simulink model "PlantaOficial"  (R2024b)
settings: Solver=ode23tb  StartTime=0.0  StopTime=39  RelTol=1e-3
values from neighbouring files (symbols this model uses):
  C1 = 1.2801    [CodigoSavePoint.m]    (also in CodigoVT.m)
  C2 = 23.99    [CodigoSavePoint.m]    (also in CodigoVT.m)
  C3 = 0.52    [CodigoSavePoint.m]    (also in CodigoVT.m)
  VelRef = 17    [CodigoSavePoint.m]    (also in CodigoVT.m = 30)
undefined symbols (not defined in the file or in its folder): EV, fractalcoef, MTR
libraries: autolibmappedmotor x2, vrlib x1, slpidlib x1, mspsensorlib x1, vehdynlibviscommon x1, vehdynlibtire x1, vehdynlibscenariocommon x1, vehdynlibsteering x1, vehdynlibdriver x1, autolibshared x1
(part 1 of 2)
settings Model: Creator=João Gabriel  LastModifiedBy=João Gabriel

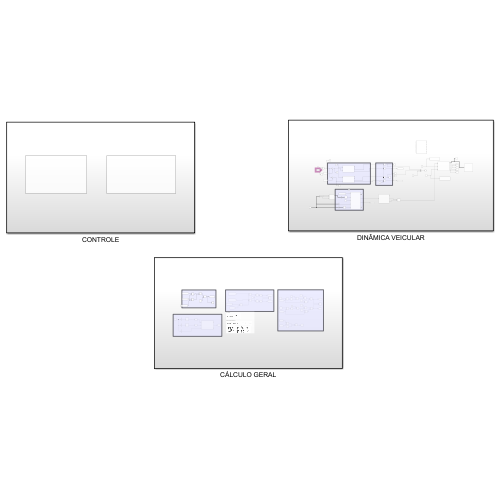
[thumbnail: Simulink's stored preview of the top-level diagram]
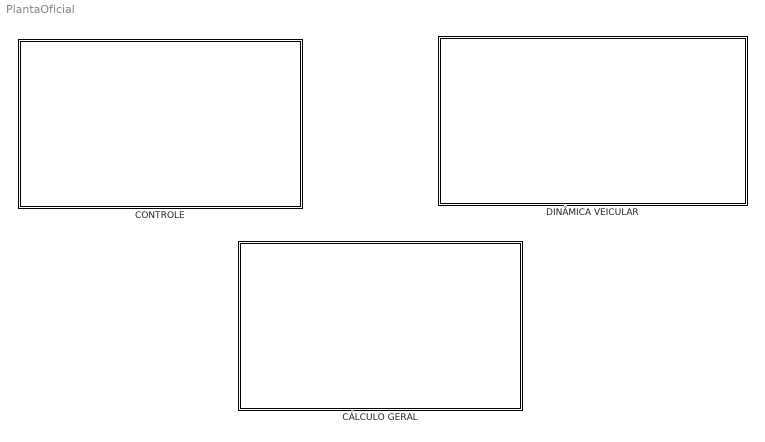
== system PlantaOficial ==
  CONTROLE : Subsystem
  CÁLCULO GERAL : Subsystem
  DINÂMICA VEICULAR : Subsystem

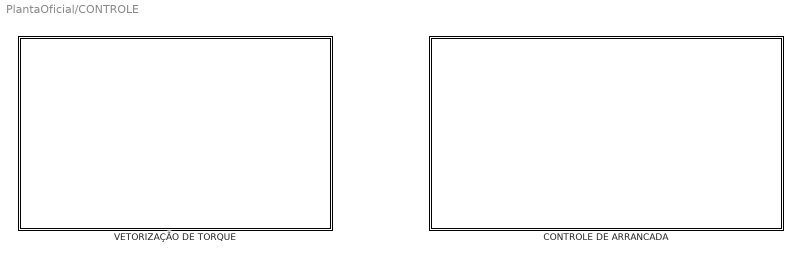
== system PlantaOficial/CONTROLE ==
  "CONTROLE DE ARRANCADA " : Subsystem
  "VETORIZAÇÃO DE TORQUE " : Subsystem

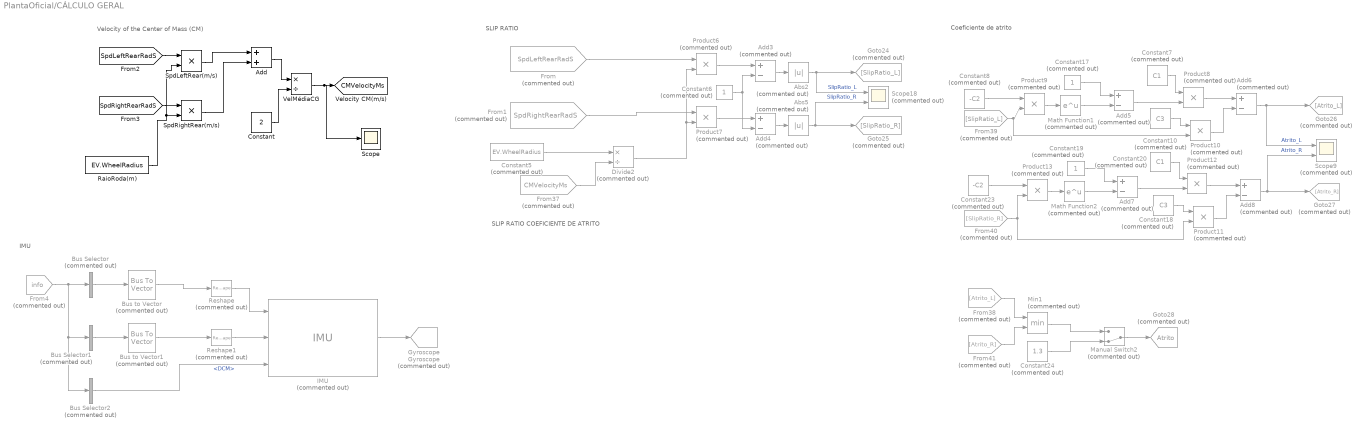
== system PlantaOficial/CÁLCULO GERAL ==
  note: IMU
  note: Velocity of the Center of Mass (CM)
  note: SLIP RATIO
  note: Coeficiente de atrito
  note: SLIP RATIO
      |
      | COEFICIENTE DE ATRITO
  Abs2 : Abs  Commented=on  SaturateOnIntegerOverflow=off
  Abs5 : Abs  Commented=on  SaturateOnIntegerOverflow=off
  Add : Sum
  Add{3..8} (6 alike) : Sum  Commented=on  Inputs=+-
  Bus Selector : BusSelector  Commented=on  OutputSignals=BdyFrm.Cg.Acc.zddot,BdyFrm.Cg.Acc.yddot,BdyFrm.Cg.Acc.xddot  OutputAsBus=on
  Bus Selector1 : BusSelector  Commented=on  OutputSignals=BdyFrm.Cg.AngVel.p,BdyFrm.Cg.AngVel.q,BdyFrm.Cg.AngVel.r  OutputAsBus=on
  Bus Selector2 : BusSelector  Commented=on  OutputSignals=BdyFrm.Cg.DCM
  Bus to Vector : BusToVector  Commented=on
  Bus to Vector1 : BusToVector  Commented=on
  Constant : Constant  Value=2
  Constant10 : Constant  Commented=on  Value=C3
  Constant17 : Constant  Commented=on
  Constant18 : Constant  Commented=on  Value=C3
  Constant19 : Constant  Commented=on
  Constant20 : Constant  Commented=on  Value=C1
  Constant23 : Constant  Commented=on  Value=-C2
  Constant24 : Constant  Commented=on  Value=1.3  VectorParams1D=off
  Constant5 : Constant  Commented=on  Value=EV.WheelRadius  VectorParams1D=off
  Constant6 : Constant  Commented=on
  Constant7 : Constant  Commented=on  Value=C1
  Constant8 : Constant  Commented=on  Value=-C2
  Divide2 : Product  Commented=on  Inputs=*/
  From : From  Commented=on  GotoTag=SpdLeftRearRadS  TagVisibility=global
  From1 : From  Commented=on  GotoTag=SpdRightRearRadS  TagVisibility=global
  From37 : From  Commented=on  GotoTag=CMVelocityMs  TagVisibility=global
  From38 : From  Commented=on  GotoTag=Atrito_L
  From39 : From  Commented=on  GotoTag=SlipRatio_L
  From4 : From  Commented=on  GotoTag=info  TagVisibility=global
  From40 : From  Commented=on  GotoTag=SlipRatio_R
  From41 : From  Commented=on  GotoTag=Atrito_R
  Goto24 : Goto  Commented=on  GotoTag=SlipRatio_L
  Goto25 : Goto  Commented=on  GotoTag=SlipRatio_R
  Goto26 : Goto  Commented=on  GotoTag=Atrito_L
  Goto27 : Goto  Commented=on  GotoTag=Atrito_R
  Goto28 : Goto  Commented=on  GotoTag=Atrito  TagVisibility=global
  "Gyroscope " : Goto  Commented=on  GotoTag=Gyroscope  TagVisibility=global
  IMU : mspsensorlib/IMU  Commented=on  DispRefFrame=NED  TemperaturePort=off  Temperature=25  MagneticFieldPort=off  MagneticFieldNED=[ 27.5550, -2.4169, -16.0849 ]  MagneticFieldENU=[ -2.4169, 27.5550, 16.0849 ]  SeedDouble=67  SimulateUsing=Interpreted execution  AccelParamsMeasurementRange=Inf  AccelParamsResolution=0  AccelParamsConstantBias=[ 0, 0, 0 ]  AccelParamsAxesMisalignment=[ 100, 0, 0; 0, 100, 0; 0, 0, 100 ]  AccelParamsNoiseDensity=[ 0, 0, 0 ]  AccelParamsBiasInstability=[ 0, 0, 0 ]  AccelParamsBiasInstabilityNumerator=fractalcoef().Numerator  AccelParamsBiasInstabilityDenominator=fractalcoef().Denominator  AccelParamsRandomWalk=[ 0, 0, 0 ]  AccelParamsNoiseType=double-sided  AccelParamsTemperatureBias=[ 0, 0, 0 ]  AccelParamsTemperatureScaleFactor=[ 0, 0, 0 ]  GyroParamsMeasurementRange=Inf  GyroParamsResolution=0  GyroParamsConstantBias=[ 0, 0, 0 ]  GyroParamsAxesMisalignment=[ 100, 0, 0; 0, 100, 0; 0, 0, 100 ]  GyroParamsAccelerationBias=[ 0, 0, 0 ]  GyroParamsNoiseDensity=[ 0, 0, 0 ]  GyroParamsBiasInstability=[ 0, 0, 0 ]  GyroParamsBiasInstabilityNumerator=fractalcoef().Numerator  GyroParamsBiasInstabilityDenominator=fractalcoef().Denominator  GyroParamsRandomWalk=[ 0, 0, 0 ]  GyroParamsNoiseType=double-sided  GyroParamsTemperatureBias=[ 0, 0, 0 ]  GyroParamsTemperatureScaleFactor=[ 0, 0, 0 ]  MagParamsMeasurementRange=Inf  MagParamsResolution=0  MagParamsConstantBias=[ 0, 0, 0 ]  MagParamsAxesMisalignment=[ 100, 0, 0; 0, 100, 0; 0, 0, 100 ]  MagParamsNoiseDensity=[ 0, 0, 0 ]  MagParamsBiasInstability=[ 0, 0, 0 ]  MagParamsBiasInstabilityNumerator=fractalcoef().Numerator  MagParamsBiasInstabilityDenominator=fractalcoef().Denominator  MagParamsRandomWalk=[ 0, 0, 0 ]  MagParamsNoiseType=double-sided  MagParamsTemperatureBias=[ 0, 0, 0 ]  MagParamsTemperatureScaleFactor=[ 0, 0, 0 ]
  Manual Switch2 : ManualSwitch  Commented=on  CurrentSetting=0
  Math Function1 : Math  Commented=on
  Math Function2 : Math  Commented=on
  Min1 : MinMax  Commented=on  Inputs=2
  Product{6..13} (8 alike) : Product  Commented=on
  RaioRoda(m) : Constant  Value=EV.WheelRadius  VectorParams1D=off
  Reshape : Reshape  Commented=on  OutputDimensionality=Customize  OutputDimensions=[1,3]
  Reshape1 : Reshape  Commented=on  OutputDimensionality=Customize  OutputDimensions=[1,3]
  Scope : Scope
  Scope18 : Scope  Commented=on  NumInputPorts=2
  Scope9 : Scope  Commented=on  NumInputPorts=2
  SpdLeftRear(m/s) : Product
  SpdRightRear(m/s) : Product
  VelMédiaCG : Product  Inputs=*/
  tag scope: CMVelocityMs=global
  wires:
  Constant6/1 -> Add3/2, Add4/2
  Add6/1 -> Scope9/1, Goto26/1  "Atrito_L"
  Abs2/1 -> Scope18/1, Goto24/1  "SlipRatio_L"
  Constant7/1 -> Product8/1
  Constant19/1 -> Add7/1
  Constant24/1 -> Manual Switch2/2
  Constant23/1 -> Product13/1
  Add4/1 -> Abs5/1
  Add3/1 -> Abs2/1
  Product11/1 -> Add8/2
  Abs5/1 -> Scope18/2, Goto25/1  "SlipRatio_R"
  Product12/1 -> Add8/1
  Product10/1 -> Add6/2
  Product8/1 -> Add6/1
  Math Function2/1 -> Add7/2
  Add7/1 -> Product12/2
  From38/1 -> Min1/1
  Constant10/1 -> Product10/1
  Math Function1/1 -> Add5/2
  Constant18/1 -> Product11/1
  From39/1 -> Product10/2, Product9/2
  Add8/1 -> Scope9/2, Goto27/1  "Atrito_R"
  Product9/1 -> Math Function1/1
  From37/1 -> Divide2/2
  Min1/1 -> Manual Switch2/1
  Constant8/1 -> Product9/1
  Constant17/1 -> Add5/1
  From41/1 -> Min1/2
  Constant5/1 -> Divide2/1
  Divide2/1 -> Product6/2, Product7/2
  Product13/1 -> Math Function2/1
  Constant20/1 -> Product12/1
  Product7/1 -> Add4/1
  Add5/1 -> Product8/2
  From40/1 -> Product13/2, Product11/2
  Product6/1 -> Add3/1
  Manual Switch2/1 -> Goto28/1
  From1/1 -> Product7/1
  From/1 -> Product6/1
  Add/1 -> VelMédiaCG/1
  RaioRoda(m)/1 -> SpdLeftRear(m/s)/2, SpdRightRear(m/s)/2
  Constant/1 -> VelMédiaCG/2
  SpdLeftRear(m/s)/1 -> Add/1
  SpdRightRear(m/s)/1 -> Add/2
  [SpdLeftRearRadS] -> SpdLeftRear(m/s)/1
  [SpdRightRearRadS] -> SpdRightRear(m/s)/1
  VelMédiaCG/1 -> Scope/1, [CMVelocityMs]
  From4/1 -> Bus Selector2/1, Bus Selector1/1, Bus Selector/1
  Bus Selector2/1 -> IMU/3  "<DCM>"
  IMU/2 -> "Gyroscope "/1
  Bus Selector/1 -> Bus to Vector/1
  Bus to Vector/1 -> Reshape/1
  Reshape/1 -> IMU/1
  Bus Selector1/1 -> Bus to Vector1/1
  Bus to Vector1/1 -> Reshape1/1
  Reshape1/1 -> IMU/2

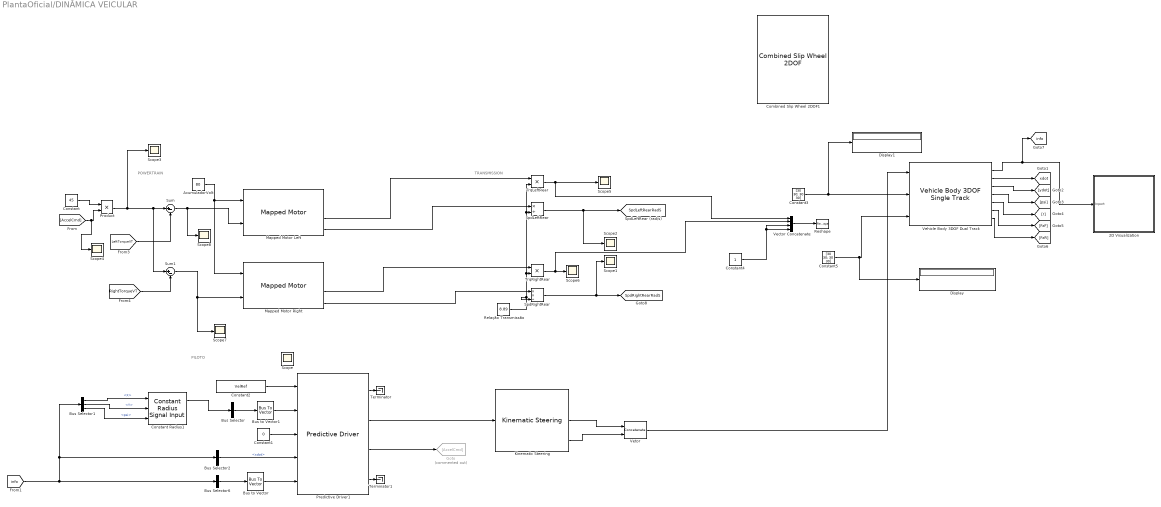
== system PlantaOficial/DINÂMICA VEICULAR ==
  note: TRANSMISSION
  note: POWERTRAIN
  note: PILOTO
  2D Visualization : Subsystem
      mask Display: image("visualization.JPG");
  AcumuladorVolt : Constant  Value=80
  Bus Selector : BusSelector  OutputSignals=XRef,YRef,PhiRef  OutputAsBus=on
  Bus Selector1 : BusSelector  OutputSignals=InertFrm.Cg.Disp.X,InertFrm.Cg.Disp.Y,InertFrm.Cg.Ang.psi
  Bus Selector2 : BusSelector  OutputSignals=BdyFrm.Cg.Vel.xdot
  Bus Selector6 : BusSelector  OutputSignals=InertFrm.Cg.Disp.X,InertFrm.Cg.Disp.Y,InertFrm.Cg.Disp.Z  OutputAsBus=on
  Bus to Vector : BusToVector
  Bus to Vector1 : BusToVector
  Combined Slip Wheel 2DOF1 : vehdynlibtire/Combined Slip Wheel 2DOF  tireType=Mid-size passenger car 235/45R18  tireParamSet=vdynPassCar.mat  vertType=Magic Formula  plySteer=on  turnslip=off  BrakeType=Disc  mu_static=.3  mu_kinetic=.2  drum_abore=0.0508  drum_a=0.123  drum_c=0.212  drum_r=0.15  drum_theta1=0  drum_theta2=126  disk_abore=.05  Rm=.177  num_pads=2  brake_p_bpt=[1 11.4736842105263 21.9473684210526 32.4210526315789 42.8947368421053 53.3684210526316 63.8421052631579 74.3157894736842 84.7894736842105 95.2631578947368 105.736842105263 116.210526315789 126.684210526316 137.157894736842 147.631578947368 158.105263157895 168.578947368421 179.052631578947 189.526315789474 200]  brake_n_bpt=[0 52.6315789473684 105.263157894737 157.894736842105 210.526315789474 263.157894736842 315.789473684211 368.421052631579 421.052631578947 473.684210526316 526.315789473684 578.947368421053 631.578947368421 684.210526315789 736.842105263158 789.473684210526 842.105263157895 894.736842105263 947.368421052632 1000]  f_brake_t=[43.4900602404453 42.5056030554862 41.5350898940194 40.5780454442085 39.6340111501808 38.7025443887544 37.7832176914519 36.8756180088306 35.9793460143796 35.0940154454303 34.2192524787115 33.3546951383474 32.4999927342521 31.6548053290159 30.8188032315107 29.991666515561 29.1730845621415 28.362755623661 27.5603864089927 26.765691687993;498.991217495636 487.695866636631 476.560505099801 465.579679307235 454.748127933653 444.060772460445 433.51270824929 423.099196101319 412.81565427025 402.657650900201 392.620896861006 382.701238955775 372.894653477208 363.197240090814 353.605216024701 344.114910546964 334.722759712992 325.425301366216 316.219170376863 307.10109410434;954.492374750826 932.886130217776 911.585920305583 890.581313170261 869.862244717126 849.419000532136 829.242198807128 809.322774193808 789.651962526121 770.221286354971 751.0225412433 732.047782773203 713.289314220164 694.739674852612 676.391628817892 658.238154578366 640.272434863842 622.48784710877 604.877954344734 587.436496520688;1409.99353200602 1378.07639379892 1346.61133551136 1315.58294703329 1284.9763615006 1254.77722860383 1224.97168936497 1195.5463522863 1166.48827078199 1137.78492180974 1109.42418562559 1081.39432659063 1053.68397496312 1026.28210961441 999.178041611083 972.361398609768 945.822110014692 919.550392851325 893.536738312604 867.771898937035;1865.49468926121 1823.26665738007 1781.63675071715 1740.58458089631 1700.09047828407 1660.13545667552 1620.7011799228 1581.76993037878 1543.32457903786 1505.34855726451 1467.82583000789 1430.74087040806 1394.07863570608 1357.82454437621 1321.96445440427 1286.48464264117 1251.37178516554 1216.61293859388 1182.19552228048 1148.10730135338;2320.9958465164 2268.45692096121 2216.66216592293 2165.58621475934 2115.20459506754 2065.49368474721 2016.43067048064 1967.99350847127 1920.16088729373 1872.91219271928 1826.22747439018 1780.08741422549 1734.47329644903 1689.36697913801 1644.75086719747 1600.60788667257 1556.92146031639 1513.67548433643 1470.85430624835 1428.44270376973;2776.49700377159 2713.64718454235 2651.68758112871 2590.58784862237 2530.31871185102 2470.8519128189 2412.16016103848 2354.21708656376 2296.9971955496 2240.47582817405 2184.62911877248 2129.43395804292 2074.86795719199 2020.9094138998 1967.53727999066 1914.73113070398 1862.47113546724 1810.73803007899 1759.51309021622 1708.77810618608;3231.99816102678 3158.8374481235 3086.71299633449 3015.58948248539 2945.43282863449 2876.21014089059 2807.88965159632 2740.44066465625 2673.83350380547 2608.03946362882 2543.03076315477 2478.78050186034 2415.26261793494 2352.4518486616 2290.32369278385 2228.85437473538 2168.02081061809 2107.80057582154 2048.17187418409 1989.11350860242;3687.49931828197 3604.02771170464 3521.73841154027 3440.59111634842 3360.54694541796 3281.56836896228 3203.61914215416 3126.66424274874 3050.66981206134 2975.60309908359 2901.43240753707 2828.12704567777 2755.6572786779 2683.9942834234 2613.11010557704 2542.97761876678 2473.57048576894 2404.8631215641 2336.83065815196 2269.44891101877;4143.00047553716 4049.21797528579 3956.76382674606 3865.59275021144 3775.66106220143 3686.92659703397 3599.34863271199 3512.88782084123 3427.50612031721 3343.16673453836 3259.83405191936 3177.4735894952 3096.05193942085 3015.5367181852 2935.89651837023 2857.10086279818 2779.12016091979 2701.92566730665 2625.48944211983 2549.78431343512;4598.50163279235 4494.40823886693 4391.78924195184 4290.59438407447 4190.77517898491 4092.28482510566 3995.07812326983 3899.11139893372 3804.34242857308 3710.73036999313 3618.23569630166 3526.82013331263 3436.44660016381 3347.079152947 3258.68293116342 3171.22410682959 3084.66983607064 2998.98821304921 2914.1482260877 2830.11971585147;5054.00279004754 4939.59850244808 4826.81465715762 4715.59601793749 4605.88929576838 4497.64305317735 4390.80761382767 4285.3349770262 4181.17873682896 4078.2940054479 3976.63734068395 3876.16667713006 3776.84126090677 3678.62158770879 3581.46934395661 3485.34735086099 ...(+2764 chars)]  NOMPRES=262000  PRESMAX=1000000  PRESMIN=10000  FNOMIN=4300  FZMAX=8600  FZMIN=100  VXLOW=1  KPUMAX=1.5  KPUMIN=-1.5  ALPMAX=1.5  ALPMIN=-1.5  CAMMAX=0.17453  CAMMIN=-0.17453  LONGVL=16.7  FxRelFreqLwrLim=200*pi  FyRelFreqLwrLim=200*pi  MyRelFreqLwrLim=100*pi  omegao=0  UNLOADED_RADIUS=0.33454  WIDTH=0.235  RIM_RADIUS=0.2286  ASPECT_RATIO=0.45  MASS=11.2  IYY=1.084  br=1e-3  GRAVITY=-9.81  zo=0  zdoto=0  BREFF=8.25094594147963  DREFF=0.260468730454265  FREFF=0.0735298544471851  Q_RE0=1.00866439868088  Q_V1=0.000760413786224011  Q_V2=0.0463384792019201  Q_FZ1=0  Q_FZ2=15.6870832810226  Q_FZ3=0  Q_FCX=0.138643970247602  Q_FCY=0.10843499565426  Q_FCY2=-0.465763352339538  PFZ1=0.69958166705601  VERTICAL_STIFFNESS=207885.061134007  VERTICAL_DAMPING=500  BOTTOM_OFFST=0.00990653336182505  BOTTOM_STIFF=1999075.87051971  Q_CAM1=86.7791723017291  Q_CAM2=259.705254231766  Q_CAM3=0.510281667378416  Q_FYS1=-20769.4728880343  Q_FYS2=-59060.183485617  Q_FYS3=89271.8260126986  LONGITUDINAL_STIFFNESS=388714.175879854  LATERAL_STIFFNESS=157087.404633332  PCFX1=0.18539229191199  PCFX2=0  PCFX3=0  PCFY1=0.163183345037677  PCFY2=0  PCFY3=0.249094918231954  Q_RA1=0.675942571700787  Q_RA2=0.73800463546164  Q_RB1=1.04487486456705  Q_RB2=-1.191763806629  PCX1=1.58523057950359  PDX1=1.0239116238178  PDX2=-0.0842405110022724  PDX3=0  PEX1=0.110312777158455  PEX2=0.313468516038146  PEX3=0  PEX4=0.0016060905760045  PKX1=21.3872544684023  PKX2=14.0006541873175  PKX3=-0.405326109653452  PHX1=0.000212599305364818  PHX2=0.00115950515263055  PVX1=1.59236164471432e-05  PVX2=0.000104321112127671  PPX1=-0.349461321276586  PPX2=0.387840040616429  PPX3=-0.0969947336569324  PPX4=0.0632271859795801  RBX1=12.7633329850276  RBX2=9.5787123658471  RBX3=0  RCX1=1.02796280922059  REX1=-0.45202516851367  REX2=-0.47304886171176  RHX1=0.000233272373115809  QSX1=-0.00788307788961443  QSX2=0.954629515459396  QSX3=0.0155855777667025  QSX4=0.125904607142414  QSX5=1.01110069703963  QSX6=20.1938577118433  QSX7=0.310818120717083  QSX8=-0.0430823751139655  QSX9=0.636494404888216  QSX10=0.142438060591663  QSX11=0.346766530036373  QSX12=0  QSX13=0  QSX14=0  PPMX1=0  PCY1=1.34299950037631  PDY1=0.878267729082195  PDY2=-0.0644597923147385  PDY3=0  PEY1=-0.809776534470972  PEY2=-0.600180598867198  PEY3=0.0991732552633487  PEY4=-6.5577974035573  PEY5=0  PKY1=-15.5714726518315  PKY2=1.73126522291751  PKY3=0.365349873517229  PKY4=1.98176755955416  PKY5=0  PKY6=-0.884005199550313  PKY7=-0.237259727611847  PHY1=-0.00183370557235628  PHY2=0.00346401302716671  PVY1=-0.00675427560163264  PVY2=0.036379218103843  PVY3=-0.163543984089166  PVY4=-0.491003349625726  PPY1=-0.62059646553185  PPY2=-0.0647824842338686  PPY3=-0.164648843290686  PPY4=0.283193909060098  PPY5=0  RBY1=10.7588809173639  RBY2=7.70420065295029  RBY3=3.40283755070691e-06  RBY4=0  RCY1=1.06691874059059  REY1=0.308244924574305  REY2=7.48775032604508e-06  RHY1=0.0118479204960415  RHY2=7.63650177161071e-06  RVY1=0.0560024425050078  RVY2=7.48487127056197e-06  RVY3=0  RVY4=98.4047026517149  RVY5=2.02759273900054  RVY6=15.7623064923347  QSY1=0.00699077564863536  QSY2=0  QSY3=0.00153535478298811  QSY4=8.55710322455322e-05  QSY5=0  QSY6=0  QSY7=0.89443879773793  QSY8=-0.403227641260894  QBZ1=11.666656027484  QBZ2=-1.30355438574485  QBZ3=0  QBZ4=0.177918305399071  QBZ5=-0.162481135068033  QBZ6=0  QBZ9=30.1445534682089  QBZ10=0  QCZ1=1.29026978207574  QDZ1=0.0886972644991399  QDZ2=-0.0058634820161856  QDZ3=0.3805597481383  QDZ4=0  QDZ6=0.00160914918118959  QDZ7=-0.00211036330862154  QDZ8=-0.13921904912557  QDZ9=0.00816585550028243  QDZ10=0  QDZ11=0  QEZ1=-2.19802254534746  QEZ2=1.01850535789165  QEZ3=0  QEZ4=0.278379679112054  QEZ5=-0.548414722765386  QHZ1=0.00148361198869669  QHZ2=0.00202017567585904  QHZ3=0.240316641332066  QHZ4=-0.210114035738085  PPZ1=-0.443927982388615  PPZ2=0  SSZ1=0.00914999585397887  SSZ2=0.0389830656052735  SSZ3=0  SSZ4=0  PDXP1=0.396718274678791  PDXP2=0  PDXP3=0  PKYP1=1.00587060633573  PDYP1=0.40483048923438  PDYP2=0  PDYP3=0  PDYP4=0  PHYP1=0.992731942067188  PHYP2=0.150352945499914  PHYP3=0  PHYP4=-3.98988682633674  PECP1=0.502379254513503  PECP2=0  QDTP1=10.0178654287947  QCRP1=0.200627747200702  QCRP2=0.0995735881599772  QBRP1=0.0997107127960717  QDRP1=1.01432910167423  QDRP2=0  aMode=2
  Constant : Constant  Value=45  VectorParams1D=off
  Constant Radius1 : vehdynlibscenariocommon/Constant Radius Signal Input  VariantControl=4  tStart=0  velRef=VelRef  velRefUnit=m/s  R=50  X_o=0  Y_o=0  psi_o=0  radialConeDist=6  ayMax=0.5  steerDir=Right  ayStop=off  use3DCones=off  aMode=2
      settings: LibrarySourceBlock=vehdynlibscenario/Constant Radius
  Constant1 : Constant  Value=0
  Constant2 : Constant  Value=VelRef  VectorParams1D=off
  Constant3 : Constant  Value=[30 30; 30 30]
  Constant4 : Constant
  Constant5 : Constant  Value=[30 30; 30 30]
  Display : Display
  Display1 : Display
  Goto : Goto  Commented=on  GotoTag=AccelCmd
  Kinematic Steering : vehdynlibsteering/Kinematic Steering  StrgType=Rack and pinion  StrgRatioType=Constant  Loc=Front  NrmlFctr=0.01  TrckWdth=1  WhlBase=1.524  Db=0  StrgRng=1.25*pi  StrgAngBpts="[-6.2832   -5.0265   -3.7699   -2.5133   -1.2566         0    1.2566    2.5133    3.7699    5.0265    6.2832]"  StrgRatioTbl=|  StrgRatio=100  PctAckIn=off  PctAck=100  PctAckTbl=ones(1,11)*100  StrgArmLngth=0.1  RckCsLngth=0.5  TieRodLngth=0.248  D=0.2  PnnRadius=0.00085818  PnnRadiusTbl="[0.0055    0.0055    0.0056    0.0057    0.0058    0.0057    0.0057    0.0057    0.0056    0.0055    0.0055]"  RodLngth=0.1  ParaArmLngth=0.9  aMode=2
      | [13.5000   13.3750   13.2500   13.1250   13.0000   13.0000   13.0000   13.1250   13.2500   13.3750   13.5000
      | ]
  Mapped Motor Left : autolibmappedmotor/Mapped Motor  w_Tmax_bp_ext=w_Tmax_bp  Tmax_w_V_ext=Tmax_w_V  w_Tmin_bp_ext=w_Tmin_bp  Tmin_w_V_ext=Tmin_w_V  port_config=Torque  param_by=Tabulated torque-speed envelope  w_t=MTR.Speed  T_t=MTR.Torque*MTR.Overpower  torque_max=.1  power_max=30  SpreadsheetTqLimitsFileName=MotorCalibrationImportData.xlsx  Tmax_w_V=[0.09 0.09 0.09;0.08 0.08 0.08;0.07 0.07 0.07;0 0 0]  w_Tmax_bp=[ 0 375 750 800 ]  V_Tmax_bp=[500 750 900]  Tmin_w_V=[-0.09 -0.09 -0.09;-0.08 -0.08 -0.08;-0.07 -0.07 -0.07;0 0 0]  w_Tmin_bp=[ 0 375 750 800 ]  V_Tmin_bp=[500 750 900]  Tc=0.05  param_loss=Single efficiency measurement  SpreadsheetLossFileName=MotorCalibrationImportData.xlsx  SpreadsheetEffFileName=MotorCalibrationImportData.xlsx  eff=100  w_eff=375  T_eff=0.08  Piron=0  Pbase=0  w_eff_bp=[-8000 -4000 0 4000 8000]  T_eff_bp=[0 0.03 0.06 0.09]  Temp_eff_bp=[233.15 293.15 373.15]  V_eff_bp=[500 700 900]  losses_table=[1.49 1.67 2.21 3.10; 0.42 0.69 1.14 2.03; 0.06 0.24 0.78 1.68; 0.42 0.69 1.14 2.03; 1.49 1.67 2.21 3.10]  losses_table_3d=cat(3,1.05*[1.49 1.67 2.21 3.10; 0.42 0.69 1.14 2.03; 0.06 0.24 0.78 1.68; 0.42 0.69 1.14 2.03; 1.49 1.67 2.21 3.10],[1.49 1.67 2.21 3.10; 0.42 0.69 1.14 2.03; 0.06 0.24 0.78 1.68; 0.42 0.69 1.14 2.03; 1.49 1.67 2.21 3.10],1.03*[1.49 1.67 2.21 3.10; 0.42 0.69 1.14 2.03; 0.06 0.24 0.78 1.68; 0.42 0.69 1.14 2.03; 1.49 1.67 2.21 3.10])  losses_table_4d=cat(4,cat(3,[1.5645 0.441 0.063 0.441 1.5645;1.7535 0.7245 0.252 0.7245 1.7535;2.3205 1.197 0.819 1.197 2.3205;3.255 2.1315 1.764 2.1315 3.255],[1.5645 0.441 0.063 0.441 1.5645;1.7535 0.7245 0.252 0.7245 1.7535;2.3205 1.197 0.819 1.197 2.3205;3.255 2.1315 1.764 2.1315 3.255],[1.5645 0.441 0.063 0.441 1.5645;1.7535 0.7245 0.252 0.7245 1.7535;2.3205 1.197 0.819 1.197 2.3205;3.255 2.1315 1.764 2.1315 3.255]),cat(3,[1.49 0.42 0.06 0.42 1.49;1.67 0.69 0.24 0.69 1.67;2.21 1.14 0.78 1.14 2.21;3.1 2.03 1.68 2.03 3.1],[1.49 0.42 0.06 0.42 1.49;1.67 0.69 0.24 0.69 1.67;2.21 1.14 0.78 1.14 2.21;3.1 2.03 1.68 2.03 3.1],[1.49 0.42 0.06 0.42 1.49;1.67 0.69 0.24 0.69 1.67;2.21 1.14 0.78 1.14 2.21;3.1 2.03 1.68 2.03 3.1]),cat(3,[1.5347 0.4326 0.0618 0.4326 1.5347;1.7201 0.7107 0.2472 0.7107 1.7201;2.2763 1.1742 0.8034 1.1742 2.2763;3.193 2.0909 1.7304 2.0909 3.193],[1.5347 0.4326 0.0618 0.4326 1.5347;1.7201 0.7107 0.2472 0.7107 1.7201;2.2763 1.1742 0.8034 1.1742 2.2763;3.193 2.0909 1.7304 2.0909 3.193],[1.5347 0.4326 0.0618 0.4326 1.5347;1.7201 0.7107 0.2472 0.7107 1.7201;2.2763 1.1742 0.8034 1.1742 2.2763;3.193 2.0909 1.7304 2.0909 3.193]))  efficiency_table=[95 95 95 95; 95 95 95 95; 95 95 95 95; 95 95 95 95; 95 95 95 95]  efficiency_table_3d=cat(3,90*ones(5,4),95*ones(5,4),92*ones(5,4))  efficiency_table_4d=cat(4,cat(3,90*ones(5,4)',90*ones(5,4)',90*ones(5,4)'),cat(3,95*ones(5,4)',95*ones(5,4)',95*ones(5,4)'),cat(3,92*ones(5,4)',92*ones(5,4)',92*ones(5,4)'))  J=5e-6  b=1e-5  omega_o=0  T_t_extended=[0.35 22.4 23.8 26.95 31.5 37.1 45.85 45.85 45.85 37.1 31.5 26.95 23.8 22.4 0.35]  w_t_extended=[-943 -942 -880 -775 -670 -565 -461 0 461 565 670 775 880 942 943]  KLossIron=0  KLossCopper=0  x_w_eff_vec=[-8000 -4000 0 4000 8000]  x_T_eff_vec=[-0.09 -0.06 -0.03 0 0.03 0.06 0.09]  x_tmp_eff_vec=[233.15 293.15 373.15]  x_V_eff_vec=[500 700 900]  x_losses_mat=[3.1 2.21 1.67 1.49 1.67 2.21 3.1;2.03 1.14 0.69 0.42 0.69 1.14 2.03;1.68 0.78 0.24 0.06 0.24 0.78 1.68;2.03 1.14 0.69 0.42 0.69 1.14 2.03;3.1 2.21 1.67 1.49 1.67 2.21 3.1]  x_losses_mat_3d=cat(3,[3.255 2.3205 1.7535 1.5645 1.7535 2.3205 3.255;2.1315 1.197 0.7245 0.441 0.7245 1.197 2.1315;1.764 0.819 0.252 0.063 0.252 0.819 1.764;2.1315 1.197 0.7245 0.441 0.7245 1.197 2.1315;3.255 2.3205 1.7535 1.5645 1.7535 2.3205 3.255],[3.1 2.21 1.67 1.49 1.67 2.21 3.1;2.03 1.14 0.69 0.42 0.69 1.14 2.03;1.68 0.78 0.24 0.06 0.24 0.78 1.68;2.03 1.14 0.69 0.42 0.69 1.14 2.03;3.1 2.21 1.67 1.49 1.67 2.21 3.1],[3.193 2.2763 1.7201 1.5347 1.7201 2.2763 3.193;2.0909 1.1742 0.7107 0.4326 0.7107 1.1742 2.0909;1.7304 0.8034 0.2472 0.0618 0.2472 0.8034 1.7304;2.0909 1.1742 0.7107 0.4326 0.7107 1.1742 2.0909;3.193 2.2763 1.7201 1.5347 1.7201 2.2763 3.193])  x_losses_mat_4d=cat(4,cat(3,[1.5645 0.441 0.063 0.441 1.5645;1.7535 0.7245 0.252 0.7245 1.7535;2.3205 1.197 0.819 1.197 2.3205;3.255 2.1315 1.764 2.1315 3.255],[1.5645 0.441 0.063 0.441 1.5645;1.7535 0.7245 0.252 0.7245 1.7535;2.3205 1.197 0.819 1.197 2.3205;3.255 2.1315 1.764 2.1315 3.255],[1.5645 0.441 0.063 0.441 1.5645;1.7535 0.7245 0.252 0.7245 1.7535;2.3205 1.197 0.819 1.197 2.3205;3.255 2.1315 1.764 2.1315 3.255]),cat(3,[1.49 0.42 0.06 0.42 1.49;1.67 0.69 0.24 0.69 1.67;2.21 1.14 0.78 1.14 2.21;3.1 2.03 1.68 2.03 3.1],[1.49 0.42 0.06 0.42 1.49;1.67 0.69 0.24 0.69 1.67;2.21 1.14 0.78 1.14 2.21;3.1 2.03 1.68 2.03 3.1],[1.49 0.42 0.06 0.42 1.49;1.67 0.69 0.24 0.69 1.67;2.21 1.14 0.78 1.14 2.21;3.1 2.03 1.68 2.03 3.1]),cat(3,[1.5347 0.4326 0.0618 0.4326 1.5347;1.7201 0.7107 0.2472 0.7107 1.7201;2.2763 1.1742 0.8034 1.1742 2.2763;3.193 2.0909 1.7304 2.0909 3.193],[1.5347 0.4326 0.0618 0.4326 1.5347;1.7201 0.7107 0.2472 0.7107 1.7201;2.2763 1.1742 0.8034 1.1742 2.2763;3.193 2.0909 1.7304 2.0909 3.193],[1.5347 0.4326 0.0618 0.4326 1.5347;1.7201 0.7107 0.2472 0.7107 1.7201;2.2763 1.1742 0.8034 1.1742 2.2763;3.193 2.0909 1.7304 2.0909 3.193]))  CalLossMapData={}  CalLossWithTempMapData={}  aMode=2  RefBlkName='autolibmappedmotor/Mapped Motor'
      settings: LibrarySourceBlock=vdynlib/Powertrain/Propulsion/Mapped Motor
  Mapped Motor Right : autolibmappedmotor/Mapped Motor  w_Tmax_bp_ext=w_Tmax_bp  Tmax_w_V_ext=Tmax_w_V  w_Tmin_bp_ext=w_Tmin_bp  Tmin_w_V_ext=Tmin_w_V  port_config=Torque  param_by=Tabulated torque-speed envelope  w_t=MTR.Speed  T_t=MTR.Torque*MTR.Overpower  torque_max=.1  power_max=30  SpreadsheetTqLimitsFileName=MotorCalibrationImportData.xlsx  Tmax_w_V=[0.09 0.09 0.09;0.08 0.08 0.08;0.07 0.07 0.07;0 0 0]  w_Tmax_bp=[ 0 375 750 800 ]  V_Tmax_bp=[500 750 900]  Tmin_w_V=[-0.09 -0.09 -0.09;-0.08 -0.08 -0.08;-0.07 -0.07 -0.07;0 0 0]  w_Tmin_bp=[ 0 375 750 800 ]  V_Tmin_bp=[500 750 900]  Tc=0.05  param_loss=Single efficiency measurement  SpreadsheetLossFileName=MotorCalibrationImportData.xlsx  SpreadsheetEffFileName=MotorCalibrationImportData.xlsx  eff=100  w_eff=375  T_eff=0.08  Piron=0  Pbase=0  w_eff_bp=[-8000 -4000 0 4000 8000]  T_eff_bp=[0 0.03 0.06 0.09]  Temp_eff_bp=[233.15 293.15 373.15]  V_eff_bp=[500 700 900]  losses_table=[1.49 1.67 2.21 3.10; 0.42 0.69 1.14 2.03; 0.06 0.24 0.78 1.68; 0.42 0.69 1.14 2.03; 1.49 1.67 2.21 3.10]  losses_table_3d=cat(3,1.05*[1.49 1.67 2.21 3.10; 0.42 0.69 1.14 2.03; 0.06 0.24 0.78 1.68; 0.42 0.69 1.14 2.03; 1.49 1.67 2.21 3.10],[1.49 1.67 2.21 3.10; 0.42 0.69 1.14 2.03; 0.06 0.24 0.78 1.68; 0.42 0.69 1.14 2.03; 1.49 1.67 2.21 3.10],1.03*[1.49 1.67 2.21 3.10; 0.42 0.69 1.14 2.03; 0.06 0.24 0.78 1.68; 0.42 0.69 1.14 2.03; 1.49 1.67 2.21 3.10])  losses_table_4d=cat(4,cat(3,[1.5645 0.441 0.063 0.441 1.5645;1.7535 0.7245 0.252 0.7245 1.7535;2.3205 1.197 0.819 1.197 2.3205;3.255 2.1315 1.764 2.1315 3.255],[1.5645 0.441 0.063 0.441 1.5645;1.7535 0.7245 0.252 0.7245 1.7535;2.3205 1.197 0.819 1.197 2.3205;3.255 2.1315 1.764 2.1315 3.255],[1.5645 0.441 0.063 0.441 1.5645;1.7535 0.7245 0.252 0.7245 1.7535;2.3205 1.197 0.819 1.197 2.3205;3.255 2.1315 1.764 2.1315 3.255]),cat(3,[1.49 0.42 0.06 0.42 1.49;1.67 0.69 0.24 0.69 1.67;2.21 1.14 0.78 1.14 2.21;3.1 2.03 1.68 2.03 3.1],[1.49 0.42 0.06 0.42 1.49;1.67 0.69 0.24 0.69 1.67;2.21 1.14 0.78 1.14 2.21;3.1 2.03 1.68 2.03 3.1],[1.49 0.42 0.06 0.42 1.49;1.67 0.69 0.24 0.69 1.67;2.21 1.14 0.78 1.14 2.21;3.1 2.03 1.68 2.03 3.1]),cat(3,[1.5347 0.4326 0.0618 0.4326 1.5347;1.7201 0.7107 0.2472 0.7107 1.7201;2.2763 1.1742 0.8034 1.1742 2.2763;3.193 2.0909 1.7304 2.0909 3.193],[1.5347 0.4326 0.0618 0.4326 1.5347;1.7201 0.7107 0.2472 0.7107 1.7201;2.2763 1.1742 0.8034 1.1742 2.2763;3.193 2.0909 1.7304 2.0909 3.193],[1.5347 0.4326 0.0618 0.4326 1.5347;1.7201 0.7107 0.2472 0.7107 1.7201;2.2763 1.1742 0.8034 1.1742 2.2763;3.193 2.0909 1.7304 2.0909 3.193]))  efficiency_table=[95 95 95 95; 95 95 95 95; 95 95 95 95; 95 95 95 95; 95 95 95 95]  efficiency_table_3d=cat(3,90*ones(5,4),95*ones(5,4),92*ones(5,4))  efficiency_table_4d=cat(4,cat(3,90*ones(5,4)',90*ones(5,4)',90*ones(5,4)'),cat(3,95*ones(5,4)',95*ones(5,4)',95*ones(5,4)'),cat(3,92*ones(5,4)',92*ones(5,4)',92*ones(5,4)'))  J=5e-6  b=1e-5  omega_o=0  T_t_extended=[0.35 22.4 23.8 26.95 31.5 37.1 45.85 45.85 45.85 37.1 31.5 26.95 23.8 22.4 0.35]  w_t_extended=[-943 -942 -880 -775 -670 -565 -461 0 461 565 670 775 880 942 943]  KLossIron=0  KLossCopper=0  x_w_eff_vec=[-8000 -4000 0 4000 8000]  x_T_eff_vec=[-0.09 -0.06 -0.03 0 0.03 0.06 0.09]  x_tmp_eff_vec=[233.15 293.15 373.15]  x_V_eff_vec=[500 700 900]  x_losses_mat=[3.1 2.21 1.67 1.49 1.67 2.21 3.1;2.03 1.14 0.69 0.42 0.69 1.14 2.03;1.68 0.78 0.24 0.06 0.24 0.78 1.68;2.03 1.14 0.69 0.42 0.69 1.14 2.03;3.1 2.21 1.67 1.49 1.67 2.21 3.1]  x_losses_mat_3d=cat(3,[3.255 2.3205 1.7535 1.5645 1.7535 2.3205 3.255;2.1315 1.197 0.7245 0.441 0.7245 1.197 2.1315;1.764 0.819 0.252 0.063 0.252 0.819 1.764;2.1315 1.197 0.7245 0.441 0.7245 1.197 2.1315;3.255 2.3205 1.7535 1.5645 1.7535 2.3205 3.255],[3.1 2.21 1.67 1.49 1.67 2.21 3.1;2.03 1.14 0.69 0.42 0.69 1.14 2.03;1.68 0.78 0.24 0.06 0.24 0.78 1.68;2.03 1.14 0.69 0.42 0.69 1.14 2.03;3.1 2.21 1.67 1.49 1.67 2.21 3.1],[3.193 2.2763 1.7201 1.5347 1.7201 2.2763 3.193;2.0909 1.1742 0.7107 0.4326 0.7107 1.1742 2.0909;1.7304 0.8034 0.2472 0.0618 0.2472 0.8034 1.7304;2.0909 1.1742 0.7107 0.4326 0.7107 1.1742 2.0909;3.193 2.2763 1.7201 1.5347 1.7201 2.2763 3.193])  x_losses_mat_4d=cat(4,cat(3,[1.5645 0.441 0.063 0.441 1.5645;1.7535 0.7245 0.252 0.7245 1.7535;2.3205 1.197 0.819 1.197 2.3205;3.255 2.1315 1.764 2.1315 3.255],[1.5645 0.441 0.063 0.441 1.5645;1.7535 0.7245 0.252 0.7245 1.7535;2.3205 1.197 0.819 1.197 2.3205;3.255 2.1315 1.764 2.1315 3.255],[1.5645 0.441 0.063 0.441 1.5645;1.7535 0.7245 0.252 0.7245 1.7535;2.3205 1.197 0.819 1.197 2.3205;3.255 2.1315 1.764 2.1315 3.255]),cat(3,[1.49 0.42 0.06 0.42 1.49;1.67 0.69 0.24 0.69 1.67;2.21 1.14 0.78 1.14 2.21;3.1 2.03 1.68 2.03 3.1],[1.49 0.42 0.06 0.42 1.49;1.67 0.69 0.24 0.69 1.67;2.21 1.14 0.78 1.14 2.21;3.1 2.03 1.68 2.03 3.1],[1.49 0.42 0.06 0.42 1.49;1.67 0.69 0.24 0.69 1.67;2.21 1.14 0.78 1.14 2.21;3.1 2.03 1.68 2.03 3.1]),cat(3,[1.5347 0.4326 0.0618 0.4326 1.5347;1.7201 0.7107 0.2472 0.7107 1.7201;2.2763 1.1742 0.8034 1.1742 2.2763;3.193 2.0909 1.7304 2.0909 3.193],[1.5347 0.4326 0.0618 0.4326 1.5347;1.7201 0.7107 0.2472 0.7107 1.7201;2.2763 1.1742 0.8034 1.1742 2.2763;3.193 2.0909 1.7304 2.0909 3.193],[1.5347 0.4326 0.0618 0.4326 1.5347;1.7201 0.7107 0.2472 0.7107 1.7201;2.2763 1.1742 0.8034 1.1742 2.2763;3.193 2.0909 1.7304 2.0909 3.193]))  CalLossMapData={}  CalLossWithTempMapData={}  aMode=2  RefBlkName='autolibmappedmotor/Mapped Motor'
      settings: LibrarySourceBlock=vdynlib/Powertrain/Propulsion/Mapped Motor
  Predictive Driver1 : vehdynlibdriver/Predictive Driver  extAccelOvr=off  extDecelOvr=off  extAccelHld=off  extDecelHld=off  extAccelZero=off  extDecelZero=off  extSteerOvr=off  extSteerHld=off  extSteerZero=off  cntrlType=PI  cntrlTypeLat=Stanley  shftType=None  coordMode=SAE J670 (Z-down)  refType=Reference pose  velUnits=m/s  angUnits=rad  gearOut=off  steerOut=off  Kp=10  Ki=5  Kff=.1  Kg=0  VehVelVec=[0 100]  KffVec=[.1 .1]  KpVec=[10 10]  KiVec=[5 5]  KgVec=[0 0]  vnom=5  Kaw=1  tauerr=.01  tau=0.1  L=3  Kpt=3000  aR=200  bR=2.5  cR=.5  g=9.81  vecPose=on  dynamMode=off  PositionGainF=2.5  PositionGainR=2.5  YawRateGain=.2  DelayGain=.2  enableDrift=off  BetaRef=20*pi/180  KpBeta=1  KpDrift=2  KdDrift=1  KpPsi=6  KOmega=30  tOmega=1  a=0.775  b=0.775  m=2016  Cy_f=25266  Cy_r=70933  I=4013  Ksteer=18  theta=0.523598776  Idl=3  Re=.3  lambda_mu=1  GearInit=0  tShift=.1  pdlVec=[0.1 0.4 0.5 0.9]  upShftTbl=[-1 12.9375 26.4375 39.9375 51.18749999999999 62.4375 72.84375 83.25;-1 16.3125 29.8125 43.3125 54.5624 65.8125 76.78125 87.75;-1 19.6875 33.1875 46.68749999999999 57.9375 69.1875 80.71875 92.25;-1 33 52.5 77.25 100.5 138.75 161.875 185]  dwnShftTbl=[-1 12.9375 26.4375 39.9375 51.18749999999999 62.4375 72.84375 83.25;-1 16.3125 29.8125 43.3125 54.5624 65.8125 76.78125 87.75;-1 19.6875 33.1875 46.68749999999999 57.9375 69.1875 80.71875 92.25;-1 33 52.5 77.25 100.5 138.75 161.875 185]  tClutch=.5  tRev=.5  tPark=120  UpGearVec="[0  1  2  3  4  5  6  7]"  DownGearVec="[1  2  3  4  5  6  7  8]"  aMode=2
  Product : Product
  Relação Transmissão : Constant  Value=8.89
  Reshape : Reshape  OutputDimensionality=Customize  OutputDimensions=[2,2]
  Scope{,1..8} (9 alike) : Scope
  SpdLeftRear : Product  Inputs=*/
  SpdRightRear : Product  Inputs=**/
  Sum : Sum  Inputs=|+-
  Sum1 : Sum  Inputs=|+-
  Terminator : Terminator
  Terminator1 : Terminator
  TrqLeftRear : Product
  TrqRightRear : Product
  Vector Concatenate : Concatenate  NumInputs=4
  Vehicle Body 3DOF Dual Track : autolibshared/Vehicle Body 3DOF Single Track  trackMode=Dual  inputMode=External forces  frontSteerMode=on  rearSteerMode=off  windMode=off  muMode=off  extFMode=off  extMMode=off  htchFMode=off  htchMMode=off  extXo=off  extpsio=off  extxdoto=off  extro=off  extYo=off  extTamb=off  extydoto=off  aMode=2  NF=2  NR=2  m=2000  a=1.4  b=1.6  h=0.35  dh=1  hh=0.2  X_o=0  xdot_o=0  CalphaMode=off  sigmaMode=on  d=0  hl=0  w=[1.4,1.4]  Cy_f=12e3  Cy_r=11e3  sigma_f=.1  sigma_r=.1  alpha_f_brk=[-.1 .1]  Cy_f_data=[-9e3 9e3]  alpha_r_brk=[-.1 .1]  Cy_r_data=[-9e3 9e3]  Y_o=0  ydot_o=0  Izz=4000  psi_o=0  r_o=0  Af=2  Cd=.3  Cl=.1  Cpm=.1  beta_w=[0 0.01:0.01:0.3]  Cs=[0:0.03:0.9]  Cym=[0 1e-6:0.01:0.3]  Pabs=101325  Tair=273  g=9.81  mu=1  xdot_tol=.01  Fznom=5000  Fxtire_sat=7e4  Fytire_sat=7e4  longOff=0  latOff=0  vertOff=0  wrapAng=off
      settings: LibrarySourceBlock=vehdynlibeom/Vehicle Body 3DOF Dual Track
  Vetor : Concatenate  ConcatenateDimension=2
  tag scope: SpdLeftRearRadS=global, SpdRightRearRadS=global, info=global, xdot=global
  wires:
  AcumuladorVolt/1 -> Mapped Motor Right/1, Mapped Motor Left/1
  Relação Transmissão/1 -> SpdRightRear/3, TrqRightRear/2, TrqLeftRear/2, SpdLeftRear/2
  Mapped Motor Right/3 -> TrqRightRear/1
  Mapped Motor Left/3 -> TrqLeftRear/1
  Mapped Motor Left/4 -> SpdLeftRear/1
  Kinematic Steering/2 -> Vetor/1
  Kinematic Steering/3 -> Vetor/2
  Vetor/1 -> Vehicle Body 3DOF Dual Track/1
  SpdRightRear/1 -> [SpdRightRearRadS], Scope1/1
  SpdLeftRear/1 -> Scope2/1, [SpdLeftRearRadS]
  Vehicle Body 3DOF Dual Track/1 -> [info], 2D Visualization/1(Inport)
  Predictive Driver1/4 -> Terminator1/1
  Predictive Driver1/1 -> Terminator/1
  Predictive Driver1/2 -> Kinematic Steering/1
  Vehicle Body 3DOF Dual Track/2 -> [xdot]
  Vehicle Body 3DOF Dual Track/3 -> [ydot]
  Vehicle Body 3DOF Dual Track/4 -> [psi]
  Vehicle Body 3DOF Dual Track/5 -> [r]
  Vehicle Body 3DOF Dual Track/6 -> [FzF]
  Vehicle Body 3DOF Dual Track/7 -> [FzR]
  [info] -> Bus Selector6/1, Bus Selector1/1, Bus Selector2/1
  Bus Selector6/1 -> Bus to Vector/1
  Bus to Vector/1 -> Predictive Driver1/5
  Bus Selector1/1 -> Constant Radius1/1  "<X>"
  Bus Selector1/2 -> Constant Radius1/2  "<Y>"
  Bus Selector1/3 -> Constant Radius1/3  "<psi>"
  Bus to Vector1/1 -> Predictive Driver1/2
  Bus Selector/1 -> Bus to Vector1/1
  Constant Radius1/1 -> Bus Selector/1
  Constant1/1 -> Predictive Driver1/3
  Bus Selector2/1 -> Predictive Driver1/4  "<xdot>"
  Constant2/1 -> Predictive Driver1/1
  Predictive Driver1/3 -> Goto/1
  Constant/1 -> Product/1
  [AccelCmd] -> Scope4/1, Product/2
  Sum/1 -> Scope8/1, Mapped Motor Left/2
  [LeftTorqueVT] -> Sum/2
  [RightTorqueVT] -> Sum1/2
  Sum1/1 -> Scope7/1, Mapped Motor Right/2
  Product/1 -> Scope3/1, Sum1/1, Sum/1
  TrqRightRear/1 -> Vector Concatenate/2, Scope6/1
  TrqLeftRear/1 -> Vector Concatenate/1, Scope5/1
  Constant3/1 -> Display1/1, Vehicle Body 3DOF Dual Track/2
  Constant4/1 -> Vector Concatenate/4, Vector Concatenate/3
  Vector Concatenate/1 -> Reshape/1
  Mapped Motor Right/4 -> SpdRightRear/1
  Constant5/1 -> Display/1, Vehicle Body 3DOF Dual Track/3

== system PlantaOficial/CONTROLE/CONTROLE DE ARRANCADA  ==

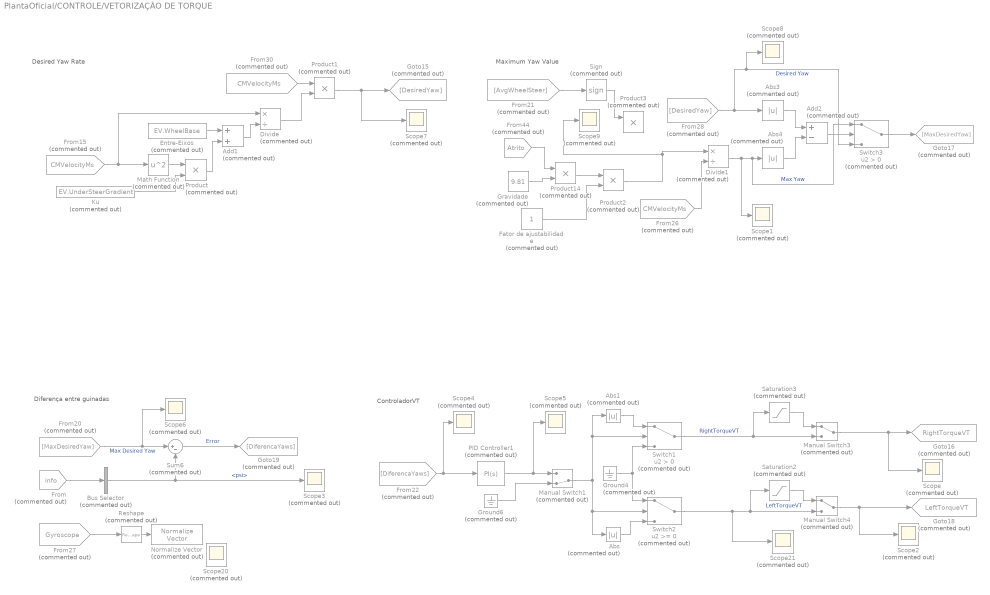
== system PlantaOficial/CONTROLE/VETORIZAÇÃO DE TORQUE  ==
  note: Desired Yaw Rate
  note: Maximum Yaw Value
  note: Diferença entre guinadas
  note: ControladorVT
  Abs{,1,3..4} (4 alike) : Abs  Commented=on  SaturateOnIntegerOverflow=off
  Add1 : Sum  Commented=on
  Add2 : Sum  Commented=on  Inputs=+-
  Bus Selector : BusSelector  Commented=on  OutputSignals=InertFrm.Cg.Ang.psi
  Divide : Product  Commented=on  Inputs=*/
  Divide1 : Product  Commented=on  Inputs=*/
  Entre-Eixos : Constant  Commented=on  Value=EV.WheelBase
  Fator de ajustabilidade : Constant  Commented=on
  From : From  Commented=on  GotoTag=info  TagVisibility=global
  From15 : From  Commented=on  GotoTag=CMVelocityMs  TagVisibility=global
  From20 : From  Commented=on  GotoTag=MaxDesiredYaw
  From21 : From  Commented=on  GotoTag=AvgWheelSteer
  From22 : From  Commented=on  GotoTag=DiferencaYaws
  From26 : From  Commented=on  GotoTag=CMVelocityMs  TagVisibility=global
  From27 : From  Commented=on  GotoTag=Gyroscope  TagVisibility=global
  From28 : From  Commented=on  GotoTag=DesiredYaw
  From30 : From  Commented=on  GotoTag=CMVelocityMs  TagVisibility=global
  From44 : From  Commented=on  GotoTag=Atrito  TagVisibility=global
  Goto15 : Goto  Commented=on  GotoTag=DesiredYaw
  Goto16 : Goto  Commented=on  GotoTag=RightTorqueVT  TagVisibility=global
  Goto17 : Goto  Commented=on  GotoTag=MaxDesiredYaw
  Goto18 : Goto  Commented=on  GotoTag=LeftTorqueVT  TagVisibility=global
  Goto19 : Goto  Commented=on  GotoTag=DiferencaYaws
  Gravidade : Constant  Commented=on  Value=9.81
  Ground4 : Ground  Commented=on
  Ground6 : Ground  Commented=on
  Ku : Constant  Commented=on  Value=EV.UnderSteerGradient
  Manual Switch1 : ManualSwitch  Commented=on  CurrentSetting=0
  Manual Switch3 : ManualSwitch  Commented=on
  Manual Switch4 : ManualSwitch  Commented=on
  Math Function : Math  Commented=on  Operator=square
  Normalize Vector : vrlib/Utilities/Normalize Vector  Commented=on  maxzero=0
  PID Controller1 : slpidlib/PID Controller  Commented=on  Controller=PI  Form=Parallel  TimeDomain=Continuous-time  UseExternalTs=off  SampleTime=-1  IntegratorMethod=Forward Euler  FilterMethod=Forward Euler  ControllerParametersSource=internal  P=278014937.203039  I=3575076642696.67  UseKiTs=off  D=-1.04450033164761  UseExternalDerivativeSource=off  N=21.9051072982779  UseFilter=on  TunerSelectOption=Transfer Function Based (PID Tuner App)  InitialConditionSource=internal  InitialConditionForIntegrator=0  InitialConditionForFilter=0  DifferentiatorICPrevScaledInput=0  ExternalReset=none  TrackingMode=off  Kt=1  LimitOutput=off  SatLimitsSource=internal  UpperSaturationLimit=inf  LowerSaturationLimit=-inf  LinearizeAsGain=on  AntiWindupMode=none  Kb=1  LimitIntegrator=off  UpperIntegratorSaturationLimit=inf  LowerIntegratorSaturationLimit=-inf  POutMin=[]  POutMax=[]  IOutMin=[]  IOutMax=[]  DOutMin=[]  DOutMax=[]  NOutMin=[]  NOutMax=[]  SumOutMin=[]  SumOutMax=[]  SaturationOutMin=[]  SaturationOutMax=[]  PParamMin=[]  PParamMax=[]  IParamMin=[]  IParamMax=[]  DParamMin=[]  DParamMax=[]  NParamMin=[]  NParamMax=[]  KbParamMin=[]  KbParamMax=[]  KtParamMin=[]  KtParamMax=[]  KbOutMin=[]  KbOutMax=[]  KtOutMin=[]  KtOutMax=[]  IntegratorOutMin=[]  IntegratorOutMax=[]  FilterOutMin=[]  FilterOutMax=[]  SumI1OutMin=[]  SumI1OutMax=[]  SumI2OutMin=[]  SumI2OutMax=[]  SumI3OutMin=[]  SumI3OutMax=[]  SumI4OutMin=[]  SumI4OutMax=[]  SumDOutMin=[]  SumDOutMax=[]  DifferentiatorOutMin=[]  DifferentiatorOutMax=[]  FilterDiffOutCoefMin=[]  FilterDiffOutCoefMax=[]  ReciprocalOutMin=[]  ReciprocalOutMax=[]  SumDenOutMin=[]  SumDenOutMax=[]  SumNumOutMin=[]  SumNumOutMax=[]  DivideOutMin=[]  DivideOutMax=[]  UdiffTsProdOutMin=[]  UdiffTsProdOutMax=[]  NTsProdOutMin=[]  NTsProdOutMax=[]  UintegralTsProdOutMin=[]  UintegralTsProdOutMax=[]  UngainTsProdOutMin=[]  UngainTsProdOutMax=[]  ClampingZeroOutDataTypeStr=Inherit: Inherit via back propagation  ClampingZeroOutMin=[]  ClampingZeroOutMax=[]  FilterDenConstantOutDataTypeStr=Inherit: Inherit via back propagation  FilterDenConstantOutMin=[]  FilterDenConstantOutMax=[]  PCopyOutDataTypeStr=Inherit: Inherit via back propagation  PCopyOutMin=[]  PCopyOutMax=[]  NCopyOutDataTypeStr=Inherit: Inherit via back propagation  NCopyOutMin=[]  NCopyOutMax=[]  IntegratorContinuousStateAttributes=''  IntegratorStateMustResolveToSignalObject=off  IntegratorRTWStateStorageClass=Auto  FilterContinuousStateAttributes=''  FilterStateMustResolveToSignalObject=off  FilterRTWStateStorageClass=Auto  ParallelPVariant=InternalParameters  IdealPVariant=Disabled  IVariant=InternalParameters  DVariant=Disabled  IntegratorVariant=Continuous  SatVariant=Disabled  AWVariant=Passthrough  PCopyVariant=Disabled  TRVariant=Disabled  FdbkBlocksVariant=Forward  IdealPFdbkVariant=Disabled  SatFdbkVariant=Disabled  DerivativeFilterVariant=Disabled  NVariant=Disabled  NCopyVariant=Disabled_SignalSpec  FilterICVariant=Disabled  IntegratorICVariant=InternalICs  ExternalResetVariant=Disabled  TRSumVariant=Passthrough  SumFdbkVariant=Disabled  SumVariant=Sum_PI  TsampFilterVariant=InternalTs  TsampNgainVariant=Passthrough  TsampIntegralVariant=Disabled_SignalSpec  ExternalSaturationOutDataTypeStr=Inherit: Same as second input  DerivativeSourceVariant=Disabled  PreIntVariant=InternalPreInt
  Product{,1..3,14} (5 alike) : Product  Commented=on
  Reshape : Reshape  Commented=on
  Saturation2 : Saturate  Commented=on  UpperLimit=11.7  LowerLimit=0
  Saturation3 : Saturate  Commented=on  UpperLimit=11.7  LowerLimit=0
  Scope{,1..9,20..21} (12 alike) : Scope  Commented=on
  Sign : Signum  Commented=on
  Sum6 : Sum  Commented=on  Inputs=|+-
  Switch1 : Switch  Commented=on  Criteria=u2 > Threshold  SaturateOnIntegerOverflow=off  InputSameDT=off
  Switch2 : Switch  Commented=on  SaturateOnIntegerOverflow=off  InputSameDT=off
  Switch3 : Switch  Commented=on  Criteria=u2 > Threshold  SaturateOnIntegerOverflow=off  InputSameDT=off
  wires:
  Product1/1 -> Scope7/1, Goto15/1
  From30/1 -> Product1/1
  Divide/1 -> Product1/2
  Math Function/1 -> Product/1
  Entre-Eixos/1 -> Add1/1
  Ku/1 -> Product/2
  Product/1 -> Add1/2
  Add1/1 -> Divide/2
  From15/1 -> Divide/1, Math Function/1
  From21/1 -> Sign/1
  From44/1 -> Product14/1
  From26/1 -> Divide1/2
  Add2/1 -> Switch3/2
  From28/1 -> Abs3/1, Scope8/1, Switch3/3  "Desired Yaw"
  Product14/1 -> Product2/1
  Divide1/1 -> Scope1/1, Switch3/1, Abs4/1  "Max Yaw"
  Sign/1 -> Product3/1
  Abs4/1 -> Add2/2
  Fator de ajustabilidade/1 -> Product2/2
  Abs3/1 -> Add2/1
  Switch3/1 -> Goto17/1
  Gravidade/1 -> Product14/2
  From20/1 -> Scope6/1, Sum6/1  "Max Desired Yaw"
  Sum6/1 -> Goto19/1  "Error"
  Manual Switch3/1 -> Scope/1, Goto16/1
  Abs/1 -> Switch2/3
  Ground4/1 -> Switch1/3, Switch2/1
  PID Controller1/1 -> Scope5/1, Manual Switch1/1
  Saturation3/1 -> Manual Switch3/1
  Switch1/1 -> Saturation3/1, Manual Switch3/2  "RightTorqueVT"
  Abs1/1 -> Switch1/1
  Manual Switch1/1 -> Abs/1, Switch2/2, Abs1/1, Switch1/2
  Ground6/1 -> Manual Switch1/2
  Manual Switch4/1 -> Scope2/1, Goto18/1
  Switch2/1 -> Saturation2/1, Manual Switch4/2, Scope21/1  "LeftTorqueVT"
  Saturation2/1 -> Manual Switch4/1
  From22/1 -> Scope4/1, PID Controller1/1
  From27/1 -> Reshape/1
  Reshape/1 -> Normalize Vector/1
  From/1 -> Bus Selector/1
  Bus Selector/1 -> Scope3/1, Sum6/2  "<psi>"
  Product2/1 -> Scope9/1, Divide1/1

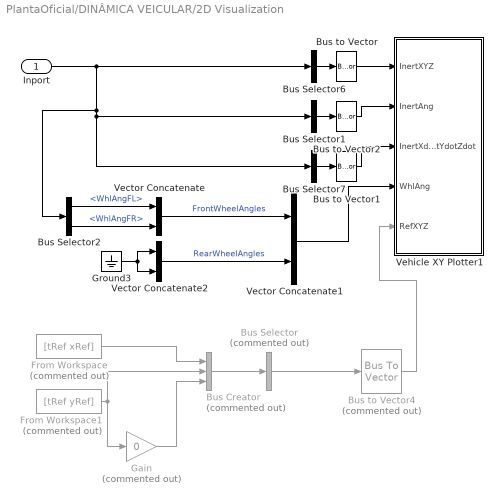
== system PlantaOficial/DINÂMICA VEICULAR/2D Visualization ==
  Inport : Inport
  Bus Creator : BusCreator  Commented=on  Inputs=3
  Bus Selector : BusSelector  Commented=on  OutputSignals=signal1,signal2,signal3  OutputAsBus=on
  Bus Selector1 : BusSelector  OutputSignals=InertFrm.Cg.Ang.phi,InertFrm.Cg.Ang.theta,InertFrm.Cg.Ang.psi  OutputAsBus=on
  Bus Selector2 : BusSelector  OutputSignals=BdyFrm.FrntAxl.Steer.WhlAngFL,BdyFrm.FrntAxl.Steer.WhlAngFR
  Bus Selector6 : BusSelector  OutputSignals=InertFrm.Geom.Disp.X,InertFrm.Geom.Disp.Y,InertFrm.Geom.Disp.Z  OutputAsBus=on
  Bus Selector7 : BusSelector  OutputSignals=InertFrm.Geom.Vel.Xdot,InertFrm.Geom.Vel.Ydot,InertFrm.Geom.Vel.Zdot  OutputAsBus=on
  Bus to Vector : BusToVector
  Bus to Vector1 : BusToVector
  Bus to Vector2 : BusToVector
  Bus to Vector4 : BusToVector  Commented=on
  From Workspace : FromWorkspace  Commented=on  VariableName=[tRef xRef]
  From Workspace1 : FromWorkspace  Commented=on  VariableName=[tRef yRef]
  Gain : Gain  Commented=on  Gain=0
  Ground3 : Ground
  Vector Concatenate : Concatenate
  Vector Concatenate1 : Concatenate
  Vector Concatenate2 : Concatenate
  Vehicle XY Plotter1 : Subsystem  mask(Vehicle XY Plotter){extRef=on, extStats=off, extTireF=off, a=2, b=2, w=2, figBorder=10, bufferSize=1024, velNorm=5, tireFNorm=1000, pltDT=0.2}
      mask prompts: extRef "Plot path reference, extRef"; extStats "Display speed, RPM and Gear"; extTireF "Display tire forces"; a "Distance to front axle from CG, a [m]:"; b "Distance to rear axle from CG, b [m]:"; w "Track width, w [m]:"; figBorder "Distance to figure borders, figBorder [m]:"; bufferSize "Path buffer sampe size, bufferSize []:"; velNorm "Velocity vector scaling, velNorm [m*s/m]:"; tireFNorm "Tire force vector scaling, tireFNorm [m/N]:"; pltDT "Plot update rate, pltDT [s]:"
      mask help:
      | This block will display a MATLAB figure which indicates the vehicle path, current position and heading velocity.
      | An optional path reference is also provided.
      mask init:
      | block = gcb;
      | if autoblkschecksimstopped(block)
      |     ParamNames = {'extRef';'extStats';'extTireF';'extTireF'};
      |     PortNames = {'RefXYZ';'Stats';'TireFx';'TireFy'};
      |     for idx=1:length(PortNames)
      |         InportOption  = {'built-in/Ground', [PortNames{idx}, ' Ground'];...
      |             'built-in/Inport',PortNames{idx}};
      |         if ~strcmp(get_param(block,ParamNames{idx}),'on')
      |             NewBlkHdl = autoblksreplaceblock(block, InportOption, 1);
      |             set_param(NewBlkHdl, 'ShowName', 'off');
      |         else
      |             autoblksreplaceblock(block, InportOption, 2);
      |         end
      |     end
      |     InportNames = {'InertXYZ';'InertAng';'InertXdotYdotZdot';'WhlAng';'RefXYZ';'Stats';'TireFx';'TireFy'};
      |     FoundNames = get_param(find_system(block, 'LookUnderMasks', 'all', 'SearchDepth', 1, 'FollowLinks', 'on', 'BlockType', 'Inport'), 'Name');
      |     [~,PortI] = intersect(InportNames, FoundNames);
      |     PortI = sort(PortI);
      |     for idx = 1:length(PortI)
      |         set_param([block, '/', InportNames{PortI(idx)}], 'Port', num2str(idx));
      |     end
      | end
      mask TypeOptions a: Vehicle XY Plotter/a
      mask TypeOptions b: Vehicle XY Plotter/b
      mask TypeOptions w: Vehicle XY Plotter/w
      mask TypeOptions figBorder: Vehicle XY Plotter/figBorder
      mask TypeOptions bufferSize: Vehicle XY Plotter/bufferSize
      mask TypeOptions velNorm: Vehicle XY Plotter/velNorm
      mask TypeOptions tireFNorm: Vehicle XY Plotter/tireFNorm
      mask DialogControl Container3 Prompt: Plot and Display Options
  wires:
  Vector Concatenate1/1 -> Vehicle XY Plotter1/4(WhlAng)
  Ground3/1 -> Vector Concatenate2/1, Vector Concatenate2/2
  Bus Selector6/1 -> Bus to Vector/1
  Vector Concatenate/1 -> Vector Concatenate1/1  "FrontWheelAngles"
  Vector Concatenate2/1 -> Vector Concatenate1/2  "RearWheelAngles"
  Bus Selector7/1 -> Bus to Vector1/1
  Bus to Vector1/1 -> Vehicle XY Plotter1/3(InertXdotYdotZdot)
  Bus to Vector/1 -> Vehicle XY Plotter1/1(InertXYZ)
  Bus to Vector2/1 -> Vehicle XY Plotter1/2(InertAng)
  Bus Selector1/1 -> Bus to Vector2/1
  Inport/1 -> Bus Selector2/1, Bus Selector7/1, Bus Selector1/1, Bus Selector6/1
  Bus to Vector4/1 -> Vehicle XY Plotter1/5(RefXYZ)
  Bus Selector/1 -> Bus to Vector4/1
  From Workspace1/1 -> Gain/1, Bus Creator/2
  Gain/1 -> Bus Creator/3
  From Workspace/1 -> Bus Creator/1
  Bus Creator/1 -> Bus Selector/1
  Bus Selector2/1 -> Vector Concatenate/1  "<WhlAngFL>"
  Bus Selector2/2 -> Vector Concatenate/2  "<WhlAngFR>"
